simulink model "PassivityBasedConfigurationSpace"  (R2018b)
settings: Solver=ode4  StartTime=0.0  StopTime=100  FixedStep=1e-3  RelTol=1e-3  EnableMultiTasking=on
settings Model: Creator=Asus  LastModifiedBy=batuhantoker
settings DataIOCC: LimitDataPoints=on
settings OptimizationCC: LifeSpan=inf
settings DebuggingCC: AllowSymbolicDim=off  SFUnexpectedBacktrackingDiag=warning  SFNoUnconditionalDefaultTransitionDiag=warning  SFExecutionAtInitializationDiag=none
settings ModelReferenceCC: PropagateSignalLabelsOutOfModel=off
settings SFSimCC: SimUseLocalCustomCode=off
settings RTWCC: RTWUseLocalCustomCode=off
settings CodeAppCC: StateflowObjectComments=on
settings GRTTargetCC: TargetLangStandard=C89/C90 (ANSI)
settings ConfigComp: CovMetricSettings=dw  CovHtmlReporting=on  CovSaveCumulativeToWorkspaceVar=on  CovSaveSingleToWorkspaceVar=on  CovExternalEMLEnable=off

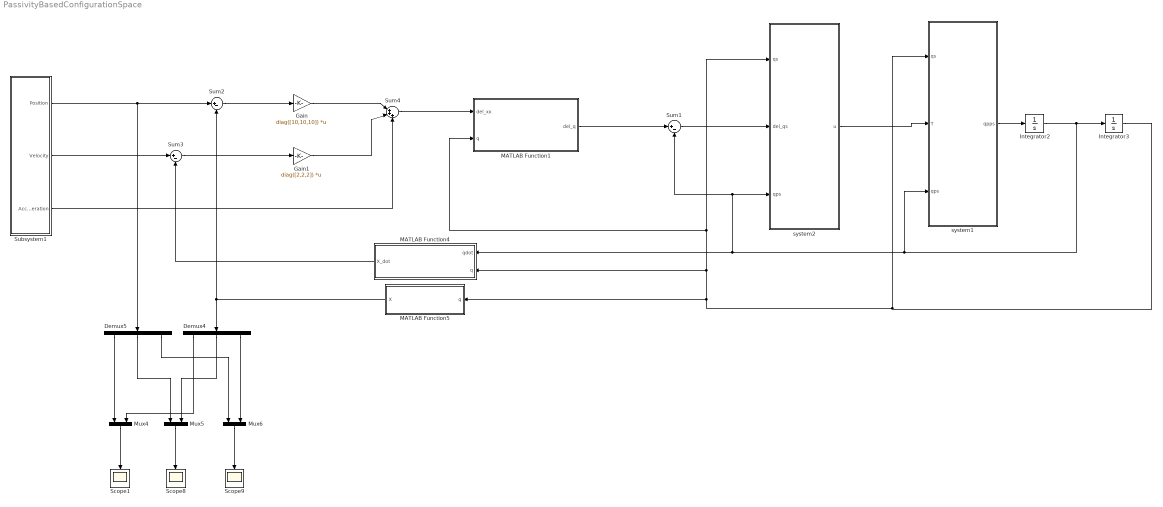
== system PassivityBasedConfigurationSpace ==
  Demux4 : Demux  Outputs=3
  Demux5 : Demux  Outputs=3
  Gain : Gain  Gain=diag([10,10,10])  Multiplication=Matrix(K*u)
  Gain1 : Gain  Gain=diag([2,2,2])  Multiplication=Matrix(K*u)
  Integrator2 : Integrator  InitialCondition=[0;0;0]
  Integrator3 : Integrator  InitialCondition=[0.001;0.001;0.001]
  MATLAB Function1 : MATLAB Function  TreatAsAtomicUnit=on
  MATLAB Function4 : MATLAB Function  TreatAsAtomicUnit=on
  MATLAB Function5 : MATLAB Function  TreatAsAtomicUnit=on
  Mux4 : Mux  Inputs=2
  Mux5 : Mux  Inputs=2
  Mux6 : Mux  Inputs=2
  Scope1 : Scope
  Scope8 : Scope
  Scope9 : Scope
  Subsystem1 : Subsystem
  Sum1 : Sum  Inputs=|+-
  Sum2 : Sum  Inputs=|+-
  Sum3 : Sum  Inputs=|+-
  Sum4 : Sum  Inputs=|+++
  system1 : MATLAB Function  TreatAsAtomicUnit=on
  system2 : MATLAB Function  TreatAsAtomicUnit=on
  wires:
  Mux5/1 -> Scope8/1
  Mux6/1 -> Scope9/1
  Demux4/1 -> Mux4/2
  Mux4/1 -> Scope1/1
  Demux5/1 -> Mux4/1
  Integrator3/1 -> system1/1(qs), system2/1(qs), MATLAB Function1/2(q), MATLAB Function4/2(q), MATLAB Function5/1(q)
  Subsystem1/1(Position) -> Sum2/1, Demux5/1
  system1/1(qpps) -> Integrator2/1
  Demux5/3 -> Mux6/1
  Demux4/2 -> Mux5/2
  Gain1/1 -> Sum4/2
  Subsystem1/3(Acceleration) -> Sum4/3
  Sum4/1 -> MATLAB Function1/1(del_xx)
  Gain/1 -> Sum4/1
  Sum2/1 -> Gain/1
  system2/1(u) -> system1/2(T)
  Sum3/1 -> Gain1/1
  Demux4/3 -> Mux6/2
  Demux5/2 -> Mux5/1
  Subsystem1/2(Velocity) -> Sum3/1
  MATLAB Function5/1(X) -> Demux4/1, Sum2/2
  MATLAB Function4/1(X_dot) -> Sum3/2
  Integrator2/1 -> MATLAB Function4/1(qdot), system2/3(qps), Sum1/2, system1/3(qps), Integrator3/1
  MATLAB Function1/1(del_q) -> Sum1/1
  Sum1/1 -> system2/2(del_qs)

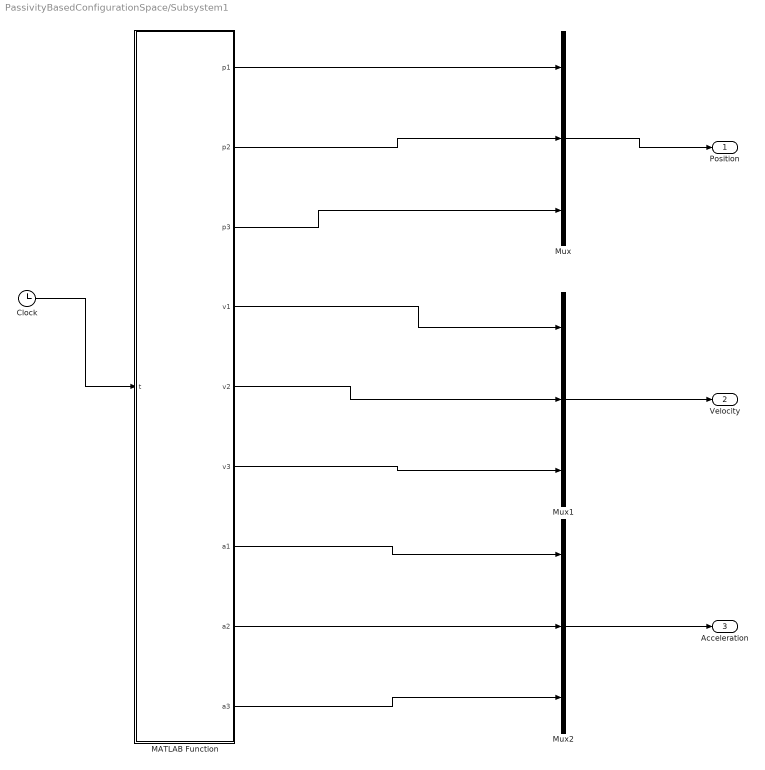
== system PassivityBasedConfigurationSpace/Subsystem1 ==
  Clock : Clock
  MATLAB Function : MATLAB Function  TreatAsAtomicUnit=on
  Mux : Mux  Inputs=3
  Mux1 : Mux  Inputs=3
  Mux2 : Mux  Inputs=3
  Position : Outport
  Velocity : Outport  Port=2
  Acceleration : Outport  Port=3
  wires:
  MATLAB Function/3(p3) -> Mux/3
  MATLAB Function/2(p2) -> Mux/2
  Mux/1 -> Position/1
  Mux1/1 -> Velocity/1
  MATLAB Function/4(v1) -> Mux1/1
  MATLAB Function/5(v2) -> Mux1/2
  MATLAB Function/1(p1) -> Mux/1
  Clock/1 -> MATLAB Function/1(t)
  MATLAB Function/6(v3) -> Mux1/3
  MATLAB Function/8(a2) -> Mux2/2
  MATLAB Function/7(a1) -> Mux2/1
  MATLAB Function/9(a3) -> Mux2/3
  Mux2/1 -> Acceleration/1

== matlab function PassivityBasedConfigurationSpace/MATLAB Function1 ==
  data: del_xx input; del_q output; q input
function del_q = Inverse_Jacobian(del_xx,q)
del_x = del_xx(1);
y_dot = del_xx(2);
z_dot = del_xx(3);
q1 = q(1);
q2 = q(2);
q3 = q(3);
l1 = 106;
l2 = 98.7;
l3 = 140.25;
del_q = (inv([- l3*cos(q2 + q3)*sin(q1) - l2*cos(q2)*sin(q1),- l3*sin(q2 + q3)*cos(q1) - l2*cos(q1)*sin(q2),-l3*sin(q2 + q3)*cos(q1);...
            l3*cos(q2 + q3)*cos(q1) + l2*cos(q1)*cos(q2),- l3*sin(q2 + q3)*sin(q1) - l2*sin(q1)*sin(q2),-l3*sin(q2 + q3)*sin(q1);...
            0,l3*cos(q2 + q3) + l2*cos(q2),l3*cos(q2 + q3)]))*[del_x;y_dot;z_dot];
q1_dot = del_q(1);
q2_dot = del_q(2);
q3_dot = del_q(3);

del_q = [q1_dot;q2_dot;q3_dot];

== matlab function PassivityBasedConfigurationSpace/Subsystem1/MATLAB Function ==
  data: t input; p1 output; p2 output; p3 output; v1 output; v2 output; v3 output; a1 output; a2 output; a3 output
function [p1,p2,p3,v1,v2,v3,a1,a2,a3] = Source(t)
p1 = 220 + 10*sin(0.1*t);
p2 = 20*cos(0.1*t);
p3 = 110;

v1 = cos(0.1*t);
v2 = -2*sin(0.1*t);
v3 = 0;

a1 = -0.1*sin(0.1*t);
a2 = -0.2*cos(0.1*t);
a3 = 0;

== matlab function PassivityBasedConfigurationSpace/system1 ==
  data: qs input; T input; qps input; qpps output
function qpps= fcn(qs, T, qps)

%inertia corilois and gravity matrix terms are taken from appendix I
q1 = qs(1);
q2 = qs(2);
q3 = qs(3);
%masses of links
m1 = 258.22;
m2 = 57.56;
m3 = 47.17;

mA = m1;
mB = m2;
mC = m3;

%inertia matirices of the links
I1 = [290212.21, 0, 0; 0, 275331.77, 0; 0, 0, 509323.35];
I2 = [7409.27 0 0; 0 52876.31 -0.01; 0 -0.01 50680.51];
I3 = [3801.21 -0.03 -0.24; -0.03 87085.96 -0.02; -0.24 -0.02 86685.11];

IA11 = I1(1,1);
IA12 = I1(1,2);
IA13 = I1(1,3);
IA21 = I1(2,1);
IA22 = I1(2,2);
IA23 = I1(2,3);
IA31 = I1(3,1);
IA32 = I1(3,2);
IA33 = I1(3,3);

IB11 = I2(1,1);
IB12 = I2(1,2);
IB13 = I2(1,3);
IB21 = I2(2,1);
IB22 = I2(2,2);
IB23 = I2(2,3);
IB31 = I2(3,1);
IB32 = I2(3,2);
IB33 = I2(3,3);

IC11 = I3(1,1);
IC12 = I3(1,2);
IC13 = I3(1,3);
IC21 = I3(2,1);
IC22 = I3(2,2);
IC23 = I3(2,3);
IC31 = I3(3,1);
IC32 = I3(3,2);
IC33 = I3(3,3);

%inertia matrix
m11 = IA33 + IB33 + IC33 + 2437.6881917025 * mB  ...
    + 4917.62782564 * mC * (cos(q2 + q3)^2 + 1.982816331884774 * cos(q2)^2 ...
    + 2.816250224596368 * cos(q2) * cos(q2 + q3)) + sin(q2 + q3) * (IC11 * sin(q2 + q3) ...
    + 2 * IC31 * cos(q2 + q3) - IC33 - sin(q2 + q3)) + sin(q2) - (IB11 - sin(q2) ...
    + 2 * IB31 * cos(q2) - 2437.6881917025 * mB * sin(q2) - IB33 * sin(q2));

m12 = -IB12 * sin(q2) - IB23 * cos(q2) - IC12 * sin(q2 + q3) - IC23 * cos(q2 + q3);
m13 = -IC12 * sin(q2 + q3) - IC23 * cos(q2 + q3);
m21 = -IB12 * sin(q2) - IB23 * cos(q2) - IC12 * sin(q2 + q3) - IC23 * cos(q2 + q3);
m22 = IB22 + IC22 + 2437.6881917025 * mB + 13849.27046844 * mC * (1.059144640569812 + cos(q3));
m23 = IC22 + 4917.62782564 * mC * (1 + 1.408125112298184 * cos(q3));
m31 = -IC12 * sin(q2 + q3) - IC23 * cos(q2 + q3);
m32 = IC22 + 4917.62782564 * mC * (1 + 1.408125112298184 * cos(q3));
m33 = IC22 + 4917.62782564 * mC;

M = [m11, m12, m13; m21, m22, m23; m31, m32, m33];

%coriolis matrix 
c11 = cos(q2)*(IB31*cos(q2)-2437.6881917025*mB*sin(q2))+2*sin(q2+q3)*(IC11*cos(q2+q3)-IC31*sin(q2+q3))...
    +2*cos(q2+q3)*(IC31*cos(q2+q3)-IC33*sin(q2+q3))+sin(q2)*(IB11*cos(q2)-IB31*sin(q2)-IB33*cos(q2))...
    -6924.635234220001*mC*(sin(q3+ 2 * q2) + 1.408125112298184 * sin(q2) * cos(q2)) ...
    - 6924.635234220001 * mC * sin(q2 + q3) * (cos(q2) + 1.420328337682881 * cos(q2 + q3));

c12 = IB23 * sin(q2) + 2 * IC23 * sin(q2 + q3) + cos(q2) * (IB31 * cos(q2)... 
    - 2437.6881917025 * mB * sin(q2)) + sin(q2 + q3) * (IC11 * cos(q2 + q3) - IC31 * sin(q2 + q3)) ...
    + cos(q2 + q3) * (IC31 * cos(q2 + q3) - IC33 * sin(q2 + q3))...
    + sin(q2) * (IB11 * cos(q2) - IB31 * sin(q2) - IB33 * cos(q2)) ...
    - IB12 * cos(q2) - 2 * IC12 * cos(q2 + q3) ...
    - 4917.62782564 * mC * (1.408125112298184 * sin(q3 + 2 * q2) ...
    + 1.982816331884774 * sin(q2) * cos(q2) + sin(q2 + q3) * cos(q2 + q3));

c13 = 2 * IC23 * sin(q2 + q3) + sin(q2 + q3) * (IC11 * cos(q2 + q3) - IC31 * sin(q2 + q3)) ...
    + cos(q2 + q3) * (IC31 * cos(q2 + q3) - IC33 * sin(q2 + q3)) - 2 * IC12 * cos(q2 + q3) ...
    - 4917.62782564 * mC * sin(q2 + q3) * (cos(q2 + q3) + 1.408125112298184 * cos(q2));

c21 = 4917.62782564 * mC * (1.408125112298184 * sin(q3 + 2 * q2) ...
    + 1.982816331884774 * sin(q2) * cos(q2) + sin(q2 + q3) * cos(q2 + q3)) ...
    - cos(q2) * (IB31 * cos(q2) - 2437.6881917025 * mB * sin(q2)) ...
    - sin(q2 + q3) * (IC11 * cos(q2 + q3) - IC31 * sin(q2 + q3)) ...
    -cos(q2 + q3) * (IC31 * cos(q2 + q3) - IC33 * sin(q2 + q3)) ...
    - sin(q2) * (IB11 * cos(q2) - IB31 * sin(q2) - IB33 * cos(q2));

c22 = -6924.63523422 * mC * sin(q3);

c23 = -13849.27046844 * mC * sin(q3);

c31 = 4917.62782564 * mC * sin(q2 + q3) * (cos(q2 + q3) + 1.408125112298184 * cos(q2))...
    - sin(q2 + q3) * (IC11 * cos(q2 + q3) - IC31 * sin(q2 + q3)) ...
    - cos(q2 + q3) * (IC31 * cos(q2 + q3) - IC33 * sin(q2 + q3));

c32 = 6924.63523422 * mC * sin(q3);

c33 = 0;

C = [c11, c12, c13; c21, c22, c23; c31, c32, c33];

%gravity matrix
g = 9810;

g1 = 0;
g2 = 49.37295 * g * (mB + 2 * mC) * cos(q2);
g3 = 70.1258 * g * mC * cos(q3);


Cqp = C * qps;
G = [g1; g2; g3];

qpps = inv(M)*(T - Cqp-G);

== matlab function PassivityBasedConfigurationSpace/system2 ==
  data: qs input; del_qs input; qps input; u output
function u= fcn(qs, del_qs, qps)

%inertia corilois and gravity matrix terms are taken from appendix I
q1 = qs(1);
q2 = qs(2);
q3 = qs(3);
%masses of links
m1 = 258.22;
m2 = 57.56;
m3 = 47.17;

mA = m1;
mB = m2;
mC = m3;

%inertia matirices of the links
I1 = [290212.21, 0, 0; 0, 275331.77, 0; 0, 0, 509323.35];
I2 = [7409.27 0 0; 0 52876.31 -0.01; 0 -0.01 50680.51];
I3 = [3801.21 -0.03 -0.24; -0.03 87085.96 -0.02; -0.24 -0.02 86685.11];

IA11 = I1(1,1);
IA12 = I1(1,2);
IA13 = I1(1,3);
IA21 = I1(2,1);
IA22 = I1(2,2);
IA23 = I1(2,3);
IA31 = I1(3,1);
IA32 = I1(3,2);
IA33 = I1(3,3);

IB11 = I2(1,1);
IB12 = I2(1,2);
IB13 = I2(1,3);
IB21 = I2(2,1);
IB22 = I2(2,2);
IB23 = I2(2,3);
IB31 = I2(3,1);
IB32 = I2(3,2);
IB33 = I2(3,3);

IC11 = I3(1,1);
IC12 = I3(1,2);
IC13 = I3(1,3);
IC21 = I3(2,1);
IC22 = I3(2,2);
IC23 = I3(2,3);
IC31 = I3(3,1);
IC32 = I3(3,2);
IC33 = I3(3,3);

%inertia matrix
m11 = IA33 + IB33 + IC33 + 2437.6881917025 * mB  ...
    + 4917.62782564 * mC * (cos(q2 + q3)^2 + 1.982816331884774 * cos(q2)^2 ...
    + 2.816250224596368 * cos(q2) * cos(q2 + q3)) + sin(q2 + q3) * (IC11 * sin(q2 + q3) ...
    + 2 * IC31 * cos(q2 + q3) - IC33 - sin(q2 + q3)) + sin(q2) - (IB11 - sin(q2) ...
    + 2 * IB31 * cos(q2) - 2437.6881917025 * mB * sin(q2) - IB33 * sin(q2));

m12 = -IB12 * sin(q2) - IB23 * cos(q2) - IC12 * sin(q2 + q3) - IC23 * cos(q2 + q3);
m13 = -IC12 * sin(q2 + q3) - IC23 * cos(q2 + q3);
m21 = -IB12 * sin(q2) - IB23 * cos(q2) - IC12 * sin(q2 + q3) - IC23 * cos(q2 + q3);
m22 = IB22 + IC22 + 2437.6881917025 * mB + 13849.27046844 * mC * (1.059144640569812 + cos(q3));
m23 = IC22 + 4917.62782564 * mC * (1 + 1.408125112298184 * cos(q3));
m31 = -IC12 * sin(q2 + q3) - IC23 * cos(q2 + q3);
m32 = IC22 + 4917.62782564 * mC * (1 + 1.408125112298184 * cos(q3));
m33 = IC22 + 4917.62782564 * mC;

M = [m11, m12, m13; m21, m22, m23; m31, m32, m33];

%coriolis matrix 
c11 = cos(q2)*(IB31*cos(q2)-2437.6881917025*mB*sin(q2))+2*sin(q2+q3)*(IC11*cos(q2+q3)-IC31*sin(q2+q3))...
    +2*cos(q2+q3)*(IC31*cos(q2+q3)-IC33*sin(q2+q3))+sin(q2)*(IB11*cos(q2)-IB31*sin(q2)-IB33*cos(q2))...
    -6924.635234220001*mC*(sin(q3+ 2 * q2) + 1.408125112298184 * sin(q2) * cos(q2)) ...
    - 6924.635234220001 * mC * sin(q2 + q3) * (cos(q2) + 1.420328337682881 * cos(q2 + q3));

c12 = IB23 * sin(q2) + 2 * IC23 * sin(q2 + q3) + cos(q2) * (IB31 * cos(q2)... 
    - 2437.6881917025 * mB * sin(q2)) + sin(q2 + q3) * (IC11 * cos(q2 + q3) - IC31 * sin(q2 + q3)) ...
    + cos(q2 + q3) * (IC31 * cos(q2 + q3) - IC33 * sin(q2 + q3))...
    + sin(q2) * (IB11 * cos(q2) - IB31 * sin(q2) - IB33 * cos(q2)) ...
    - IB12 * cos(q2) - 2 * IC12 * cos(q2 + q3) ...
    - 4917.62782564 * mC * (1.408125112298184 * sin(q3 + 2 * q2) ...
    + 1.982816331884774 * sin(q2) * cos(q2) + sin(q2 + q3) * cos(q2 + q3));

c13 = 2 * IC23 * sin(q2 + q3) + sin(q2 + q3) * (IC11 * cos(q2 + q3) - IC31 * sin(q2 + q3)) ...
    + cos(q2 + q3) * (IC31 * cos(q2 + q3) - IC33 * sin(q2 + q3)) - 2 * IC12 * cos(q2 + q3) ...
    - 4917.62782564 * mC * sin(q2 + q3) * (cos(q2 + q3) + 1.408125112298184 * cos(q2));

c21 = 4917.62782564 * mC * (1.408125112298184 * sin(q3 + 2 * q2) ...
    + 1.982816331884774 * sin(q2) * cos(q2) + sin(q2 + q3) * cos(q2 + q3)) ...
    - cos(q2) * (IB31 * cos(q2) - 2437.6881917025 * mB * sin(q2)) ...
    - sin(q2 + q3) * (IC11 * cos(q2 + q3) - IC31 * sin(q2 + q3)) ...
    -cos(q2 + q3) * (IC31 * cos(q2 + q3) - IC33 * sin(q2 + q3)) ...
    - sin(q2) * (IB11 * cos(q2) - IB31 * sin(q2) - IB33 * cos(q2));

c22 = -6924.63523422 * mC * sin(q3);

c23 = -13849.27046844 * mC * sin(q3);

c31 = 4917.62782564 * mC * sin(q2 + q3) * (cos(q2 + q3) + 1.408125112298184 * cos(q2))...
    - sin(q2 + q3) * (IC11 * cos(q2 + q3) - IC31 * sin(q2 + q3)) ...
    - cos(q2 + q3) * (IC31 * cos(q2 + q3) - IC33 * sin(q2 + q3));

c32 = 6924.63523422 * mC * sin(q3);

c33 = 0;

C = [c11, c12, c13; c21, c22, c23; c31, c32, c33];

%gravity matrix
g = 9810;

g1 = 0;
g2 = 49.37295 * g * (mB + 2 * mC) * cos(q2);
g3 = 70.1258 * g * mC * cos(q3);


Cqp = C * qps;
G = [g1; g2; g3];

u = M*del_qs + Cqp + G;

== matlab function PassivityBasedConfigurationSpace/MATLAB Function4 ==
  data: qdot input; q input; X_dot output
function X_dot = Motion_Level_Kinematics(qdot,q)
q1 = q(1);
q2 = q(2);
q3 = q(3);
qdot1 = qdot(1);
qdot2 = qdot(2);
qdot3 = qdot(3);
l1 = 106;
l2 = 98.7;
l3 = 140.25;
ee_dot = [- l3*cos(q2 + q3)*sin(q1) - l2*cos(q2)*sin(q1),- l3*sin(q2 + q3)*cos(q1) - l2*cos(q1)*sin(q2),-l3*sin(q2 + q3)*cos(q1);...
            l3*cos(q2 + q3)*cos(q1) + l2*cos(q1)*cos(q2),- l3*sin(q2 + q3)*sin(q1) - l2*sin(q1)*sin(q2),-l3*sin(q2 + q3)*sin(q1);...
            0,l3*cos(q2 + q3) + l2*cos(q2),l3*cos(q2 + q3)]*[qdot1;qdot2;qdot3];
x_dot = ee_dot(1);
y_dot = ee_dot(2);
z_dot = ee_dot(3);

X_dot = [x_dot;y_dot;z_dot];

== matlab function PassivityBasedConfigurationSpace/MATLAB Function5 ==
  data: q input; X output
function X = Forward_Kinematics(q)
q1 = q(1);
q2 = q(2);
q3 = q(3);
l1 = 106;
l2 = 98.7;
l3 = 140.25;
x =  l3*cos(q1)*cos(q2 + q3) + l2*cos(q1)*cos(q2);
y = l3*sin(q1)*cos(q2 + q3) + l2*sin(q1)*cos(q2);
z = l3*sin(q2 +q3) + l2*sin(q2) + l1;

X = [x;y;z];
